simulink subsystem "IdealFixedGearTransmission"  (R2025b)
settings: Solver=VariableStepAuto  StartTime=0.0  StopTime=10.0  RelTol=1e-3
undefined symbols (not defined in the file): PlntDriveshftDamp, PlntDriveshftStiff, PlntTransEffTempBpt, PlntTransGearRatioVect
libraries: autolibsharedcoupling x1, autolibsharedtransfixedgear x1
settings Model: ModifiedByFormat=The MathWorks, Inc.  Creator=The MathWorks, Inc.  LastModifiedBy=The MathWorks, Inc.
settings SolverCC: MaxZcPerStep=1.0
settings ModelReferenceCC: EnableRefExpFcnMdlSchedulingChecks=on
settings RTWCC: GPUComputeCapability=3.5

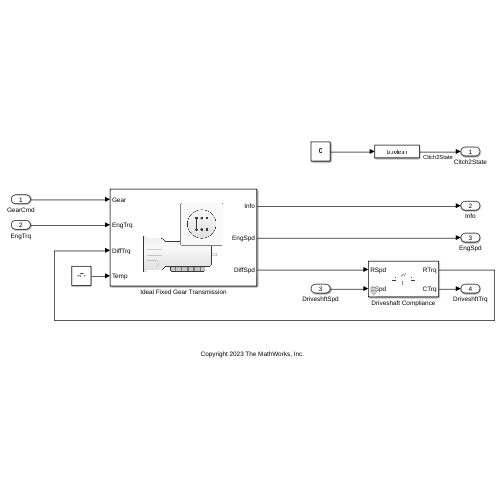
[thumbnail: Simulink's stored preview of the top-level diagram]
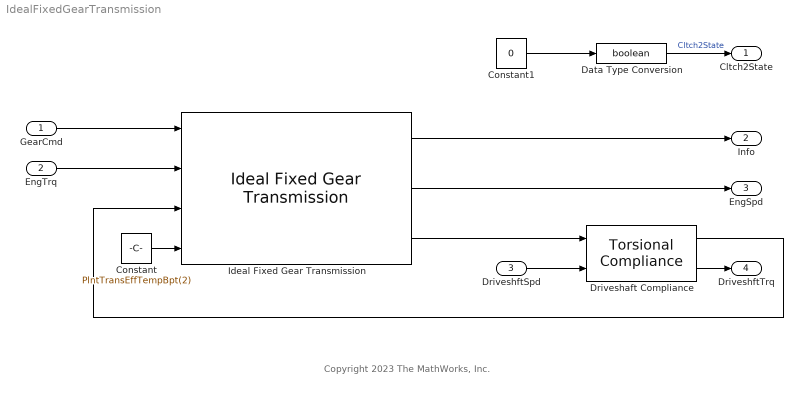
== system IdealFixedGearTransmission ==
  note: Copyright 2023 The MathWorks, Inc.
  GearCmd : Inport
  EngTrq : Inport  Port=2
  DriveshftSpd : Inport  Port=3
  Constant : Constant  Value=PlntTransEffTempBpt(2)  SampleTime=-1
  Constant1 : Constant  Value=0  SampleTime=-1
  Data Type Conversion : DataTypeConversion  OutDataTypeStr=boolean  SaturateOnIntegerOverflow=off  RndMeth=Floor
  Driveshaft Compliance : autolibsharedcoupling/Torsional Compliance  port_config=Simulink  extInfo=off  k=PlntDriveshftStiff  b=PlntDriveshftDamp  theta_o=PlntDriveshftInitDeflect  domega_o=PlntDriveshftInitVel  omega_c=PlntDriveshftDampCutoffFreq  blkID=0  aMode=6
  Ideal Fixed Gear Transmission : autolibsharedtransfixedgear/Ideal Fixed Gear Transmission  VariantControl=0  TransEffModelPopup=Gear, input torque, input speed, and temperature  gearInterp=Linear point-slope  G=PlntTransGearNumVect  Trq_bpts=PlntTransEffTrqBpt  omega_bpts=PlntTransEffSpdBpt  Temp_bpts=PlntTransEffTempBpt  N=PlntTransGearRatioVect  Jout=PlntTransInertiaVect  bout=PlntTransDampVect  eta=PlntTransEffVect  eta_tbl=PlntTransEffTbl  G_o=PlntTransInitGear  omega_o=PlntTransInitOutVel  omegaN_o=PlntTransInitNtrlInVel  tau_s=PlntTransShftTimeCnst  maxAbsSpd=5e3  aMode=6
  Cltch2State : Outport  VectorParamsAs1DForOutWhenUnconnected=off
  Info : Outport  Port=2  VectorParamsAs1DForOutWhenUnconnected=off
  EngSpd : Outport  Port=3  VectorParamsAs1DForOutWhenUnconnected=off
  DriveshftTrq : Outport  Port=4  VectorParamsAs1DForOutWhenUnconnected=off
  wires:
  DriveshftSpd/1 -> Driveshaft Compliance/2
  EngTrq/1 -> Ideal Fixed Gear Transmission/2
  GearCmd/1 -> Ideal Fixed Gear Transmission/1
  Ideal Fixed Gear Transmission/1 -> Info/1
  Driveshaft Compliance/1 -> Ideal Fixed Gear Transmission/3
  Ideal Fixed Gear Transmission/3 -> Driveshaft Compliance/1
  Constant1/1 -> Data Type Conversion/1
  Constant/1 -> Ideal Fixed Gear Transmission/4
  Driveshaft Compliance/2 -> DriveshftTrq/1
  Ideal Fixed Gear Transmission/2 -> EngSpd/1
  Data Type Conversion/1 -> Cltch2State/1  "Cltch2State"
